simulink model "NewModuleTry_cs"  (Simulink 8.4)
settings: Solver=ode5  SolverMode=SingleTasking  StartTime=0.0  StopTime=inf  FixedStep=1/100  RelTol=1e-3
PreLoadFcn:
  | mbxruntime.callbacks.PreLoadFcn(bdroot);
PostLoadFcn:
  | mbxruntime.callbacks.PostLoadFcn(bdroot);
InitFcn:
  | mbxruntime.callbacks.InitFcn(bdroot);
StartFcn:
  | mbxruntime.callbacks.StartFcn(bdroot);
StopFcn:
  | mbxruntime.callbacks.StopFcn(bdroot);
undefined symbols (not defined in the file or in its folder): dfreq, gray, InitImageOutputDir, Rec, SDTV, strel
libraries: simulink x41, PreScanSimulinkLibrary x15, visiontextngfix x15, simulink_extras x12, visionconversions x3, PreScanUsefulBlocks x3, visionsinks x2, visionstatistics x1, visionmorphops x1, visionanalysis x1, simulink_need_slupdate x1
(part 4 of 7)

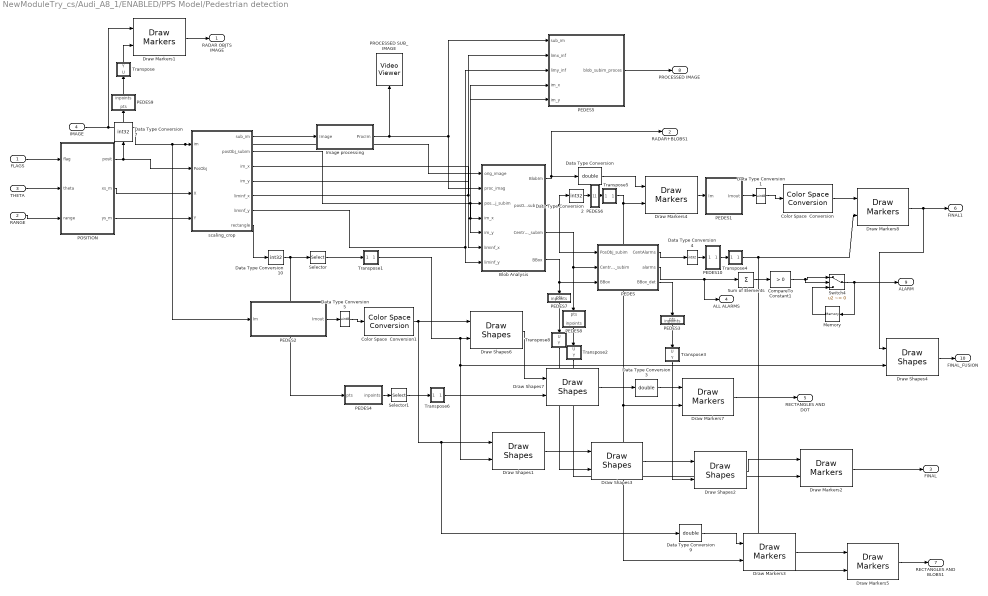
== system NewModuleTry_cs/Audi_A8_1/ENABLED/PPS Model/Pedestrian detection ==
  FLAGS : Inport  OutDataTypeStr=boolean
  RANGE : Inport  Port=2  PortDimensions=TISdet
  THETA : Inport  Port=3
  IMAGE : Inport  Port=4  OutDataTypeStr=uint8  PortDimensions=[375 500]
  Blob Analysis : Subsystem
  Color Space  Conversion : visionconversions/Color Space  Conversion  conversion=Obsolete  conversionActive=Y'CbCr to R'G'B'  wp_str=D65  rec=Rec. 601 (SDTV)  sys=1125/60/2:1  imagePorts=One multidimensional signal
  Color Space  Conversion1 : visionconversions/Color Space  Conversion  conversion=Obsolete  conversionActive=Y'CbCr to R'G'B'  wp_str=D65  rec=Rec. 601 (SDTV)  sys=1125/60/2:1  imagePorts=One multidimensional signal
  CompareTo Constant1 : simulink/Logic and Bit Operations/Compare To Constant  relop=>  const=0  OutDataTypeStr=uint8
  Data Type Conversion : DataTypeConversion  OutDataTypeStr=double
  Data Type Conversion1 : DataTypeConversion  OutDataTypeStr=uint8
  Data Type Conversion{2,4,7,10} (4 alike) : DataTypeConversion  OutDataTypeStr=int32
  Data Type Conversion3 : DataTypeConversion  OutDataTypeStr=double
  Data Type Conversion5 : DataTypeConversion  OutDataTypeStr=uint8
  Data Type Conversion9 : DataTypeConversion  OutDataTypeStr=double
  Draw Markers1 : visiontextngfix/Draw Markers  shape=Circle  size=6  fill=on  fillClrSource=Specify via dialog  display=White  intensity=200  color=[200 255 100]  opacity=1  viewport=Entire image  antialiasing=on  inType=Obsolete  imagePorts=One multidimensional signal  prodOutputMode=Binary point scaling  prodOutputWordLength=32  prodOutputFracLength=14  memoryMode=Specify word length  memoryWordLength=16  memoryFracLength=14  roundingMode=Floor  overflowMode=off
  Draw Markers2 : visiontextngfix/Draw Markers  shape=X-mark  size=3  fill=on  fillClrSource=Specify via dialog  display=White  intensity=200  color=[200 255 100]  opacity=0.9  viewport=Entire image  antialiasing=on  inType=Obsolete  imagePorts=One multidimensional signal  prodOutputMode=Binary point scaling  prodOutputWordLength=32  prodOutputFracLength=14  memoryMode=Specify word length  memoryWordLength=16  memoryFracLength=14  roundingMode=Floor  overflowMode=off
  Draw Markers3 : visiontextngfix/Draw Markers  shape=Circle  size=6  fill=on  fillClrSource=Specify via dialog  display=White  intensity=200  color=[255 0 0]  opacity=0.9  viewport=Entire image  antialiasing=on  inType=Obsolete  imagePorts=One multidimensional signal  prodOutputMode=Binary point scaling  prodOutputWordLength=32  prodOutputFracLength=14  memoryMode=Specify word length  memoryWordLength=16  memoryFracLength=14  roundingMode=Floor  overflowMode=off
  Draw Markers4 : visiontextngfix/Draw Markers  shape=Circle  size=6  fill=on  fillClrSource=Specify via dialog  display=White  intensity=200  color=[200 255 100]  opacity=0.9  viewport=Entire image  antialiasing=on  inType=Obsolete  imagePorts=One multidimensional signal  prodOutputMode=Binary point scaling  prodOutputWordLength=32  prodOutputFracLength=14  memoryMode=Specify word length  memoryWordLength=16  memoryFracLength=14  roundingMode=Floor  overflowMode=off
  Draw Markers5 : visiontextngfix/Draw Markers  shape=Circle  size=6  fill=on  fillClrSource=Specify via dialog  display=User-specified value  intensity=200  color=[255 0 0]  opacity=1  viewport=Entire image  antialiasing=on  inType=Obsolete  imagePorts=One multidimensional signal  prodOutputMode=Binary point scaling  prodOutputWordLength=32  prodOutputFracLength=14  memoryMode=Specify word length  memoryWordLength=16  memoryFracLength=14  roundingMode=Floor  overflowMode=off
  Draw Markers7 : visiontextngfix/Draw Markers  shape=Circle  size=6  fill=on  fillClrSource=Specify via dialog  display=White  intensity=200  color=[200 255 100]  opacity=0.9  viewport=Entire image  antialiasing=on  inType=Obsolete  imagePorts=One multidimensional signal  prodOutputMode=Binary point scaling  prodOutputWordLength=32  prodOutputFracLength=14  memoryMode=Specify word length  memoryWordLength=16  memoryFracLength=14  roundingMode=Floor  overflowMode=off
  Draw Markers8 : visiontextngfix/Draw Markers  shape=Circle  size=6  fill=on  fillClrSource=Specify via dialog  display=User-specified value  intensity=200  color=[255 0 0]  opacity=1  viewport=Entire image  antialiasing=on  inType=Obsolete  imagePorts=One multidimensional signal  prodOutputMode=Binary point scaling  prodOutputWordLength=32  prodOutputFracLength=14  memoryMode=Specify word length  memoryWordLength=16  memoryFracLength=14  roundingMode=Floor  overflowMode=off
  Draw Shapes1 : visiontextngfix/Draw Shapes  shape=Rectangles  fill=off  lineWidth=1  fillClrSource=Specify via dialog  display=White  intensity=200  color=[255 0 0]  opacity=0.5  viewport=Entire image  antialiasing=off  inType=Obsolete  imagePorts=One multidimensional signal  prodOutputMode=Binary point scaling  prodOutputWordLength=32  prodOutputFracLength=14  memoryMode=Specify word length  memoryWordLength=16  memoryFracLength=14  roundingMode=Floor  overflowMode=off
  Draw Shapes2 : visiontextngfix/Draw Shapes  shape=Rectangles  fill=on  lineWidth=1  fillClrSource=Specify via dialog  display=White  intensity=200  color=[255 0 0]  opacity=0.5  viewport=Entire image  antialiasing=off  inType=Obsolete  imagePorts=One multidimensional signal  prodOutputMode=Binary point scaling  prodOutputWordLength=32  prodOutputFracLength=14  memoryMode=Specify word length  memoryWordLength=16  memoryFracLength=14  roundingMode=Floor  overflowMode=off
  Draw Shapes3 : visiontextngfix/Draw Shapes  shape=Rectangles  fill=off  lineWidth=1  fillClrSource=Specify via dialog  display=User-specified value  intensity=200  color=[255 0 0]  opacity=0.5  viewport=Entire image  antialiasing=off  inType=Obsolete  imagePorts=One multidimensional signal  prodOutputMode=Binary point scaling  prodOutputWordLength=32  prodOutputFracLength=14  memoryMode=Specify word length  memoryWordLength=16  memoryFracLength=14  roundingMode=Floor  overflowMode=off
  Draw Shapes4 : visiontextngfix/Draw Shapes  shape=Rectangles  fill=off  lineWidth=1  fillClrSource=Specify via dialog  display=White  intensity=200  color=[255 0 0]  opacity=0.5  viewport=Entire image  antialiasing=off  inType=Obsolete  imagePorts=One multidimensional signal  prodOutputMode=Binary point scaling  prodOutputWordLength=32  prodOutputFracLength=14  memoryMode=Specify word length  memoryWordLength=16  memoryFracLength=14  roundingMode=Floor  overflowMode=off
  Draw Shapes6 : visiontextngfix/Draw Shapes  shape=Rectangles  fill=off  lineWidth=1  fillClrSource=Specify via dialog  display=User-specified value  intensity=200  color=[255 0 0]  opacity=0.6  viewport=Entire image  antialiasing=off  inType=Obsolete  imagePorts=One multidimensional signal  prodOutputMode=Binary point scaling  prodOutputWordLength=32  prodOutputFracLength=14  memoryMode=Specify word length  memoryWordLength=16  memoryFracLength=15  roundingMode=Floor  overflowMode=off
  Draw Shapes7 : visiontextngfix/Draw Shapes  shape=Rectangles  fill=on  lineWidth=1  fillClrSource=Specify via dialog  display=White  intensity=200  color=[255 0 0]  opacity=0.5  viewport=Entire image  antialiasing=off  inType=Obsolete  imagePorts=One multidimensional signal  prodOutputMode=Binary point scaling  prodOutputWordLength=32  prodOutputFracLength=14  memoryMode=Specify word length  memoryWordLength=16  memoryFracLength=14  roundingMode=Floor  overflowMode=off
  Image processing : Subsystem
  Memory : Memory
  PEDES : MATLAB Function  TreatAsAtomicUnit=on
  PEDES1 : MATLAB Function  TreatAsAtomicUnit=on
  PEDES10 : MATLAB Function  TreatAsAtomicUnit=on
  PEDES2 : MATLAB Function  TreatAsAtomicUnit=on
  PEDES3 : MATLAB Function  TreatAsAtomicUnit=on
  PEDES4 : MATLAB Function  TreatAsAtomicUnit=on
  PEDES5 : MATLAB Function  TreatAsAtomicUnit=on
  PEDES6 : MATLAB Function  TreatAsAtomicUnit=on
  PEDES7 : MATLAB Function  TreatAsAtomicUnit=on
  PEDES8 : MATLAB Function  TreatAsAtomicUnit=on
  PEDES9 : MATLAB Function  TreatAsAtomicUnit=on
  POSITION : MATLAB Function  TreatAsAtomicUnit=on
  PROCESSED SUB_IMAGE : visionsinks/Video Viewer  inputType=Obsolete7b  imagePorts=One multidimensional signal  useColorMap=off  colormapValue=gray(256)  specRange=off  minInputVal=0  maxInputVal=255  FigPos=[662 991 500 324]  AxisZoom=on  trueSizedOnce=off  OpenAtMdlStart=on  DefaultConfigurationName=vipscopes.VideoViewerScopeCfg
  Selector : Selector  InputPortWidth=4  Indices=[2, 1, 4, 3]
  Selector1 : Selector  InputPortWidth=4  Indices=[2, 1, 4, 3]
  Sum of Elements : Sum  Inputs=+
  Switch4 : Switch  Criteria=u2 ~= 0
  Transpose : Subsystem
  Transpose1 : Subsystem
  Transpose2 : Subsystem
  Transpose3 : Subsystem
  Transpose4 : Subsystem
  Transpose5 : Subsystem
  Transpose6 : Subsystem
  Transpose8 : Subsystem
  scaling_crop : MATLAB Function  TreatAsAtomicUnit=on
  RADAR OBJTS IMAGE : Outport
  RADAR+BLOBS1 : Outport  Port=2
  FINAL : Outport  Port=3
  ALL ALARMS : Outport  Port=4
  RECTANGLES AND DOT : Outport  Port=5
  FINAL1 : Outport  Port=6
  RECTANGLES AND BLOBS1 : Outport  Port=7
  PROCESSED IMAGE : Outport  Port=8
  ALARM : Outport  Port=9
  FINAL_FUSION : Outport  Port=10
  wires:
  THETA/1 -> POSITION/2(theta)
  FLAGS/1 -> POSITION/1(flag)
  RANGE/1 -> POSITION/3(range)
  Blob Analysis/1(BlobIm) -> RADAR+BLOBS1/1, Data Type Conversion/1
  Blob Analysis/3(Centroid_subim) -> PEDES/2(Centroid_subim), PEDES8/1(pts)
  PEDES/2(alarms) -> ALL ALARMS/1, Sum of Elements/1
  PEDES/1(CentAlarms) -> Data Type Conversion4/1
  Blob Analysis/4(BBox) -> PEDES/3(BBox), PEDES7/1(pts)
  Draw Markers4/1 -> PEDES1/1(Im)
  Data Type Conversion4/1 -> PEDES10/1(pts)
  Color Space  Conversion/1 -> Draw Markers8/1
  PEDES1/1(Imout) -> Data Type Conversion1/1
  Data Type Conversion1/1 -> Color Space  Conversion/1
  Data Type Conversion2/1 -> PEDES6/1(pts)
  Switch4/1 -> Memory/1, ALARM/1
  Memory/1 -> Switch4/3
  Sum of Elements/1 -> CompareTo Constant1/1
  CompareTo Constant1/1 -> Switch4/1, Switch4/2
  Blob Analysis/2(posObj_subim1) -> Data Type Conversion2/1, PEDES/1(PosObj_subim)
  scaling_crop/6(liminf_y) -> PEDES5/3(limy_inf), Blob Analysis/7(liminf_y)
  scaling_crop/7(rectangle) -> Data Type Conversion10/1
  PEDES2/1(Imout) -> Data Type Conversion5/1
  Data Type Conversion5/1 -> Color Space  Conversion1/1
  Color Space  Conversion1/1 -> Draw Shapes6/1, Data Type Conversion9/1, Draw Shapes1/1
  Draw Shapes6/1 -> Draw Shapes7/1
  Draw Shapes7/1 -> Data Type Conversion3/1
  Draw Markers7/1 -> RECTANGLES AND DOT/1
  Draw Shapes1/1 -> Draw Shapes3/1
  Draw Shapes3/1 -> Draw Shapes2/1
  Draw Shapes2/1 -> Draw Markers2/1
  Draw Markers3/1 -> Draw Markers5/1
  Draw Markers5/1 -> RECTANGLES AND BLOBS1/1
  PEDES5/1(blob_subim_proces) -> PROCESSED IMAGE/1
  Draw Markers8/1 -> FINAL1/1, Draw Shapes4/1
  Draw Shapes4/1 -> FINAL_FUSION/1
  Data Type Conversion7/1 -> PEDES9/1(pts)
  POSITION/2(xs_m) -> scaling_crop/3(X)
  Draw Markers1/1 -> RADAR OBJTS IMAGE/1
  POSITION/3(ys_m) -> scaling_crop/4(Y)
  POSITION/1(posit) -> scaling_crop/2(PosObj), Data Type Conversion7/1
  IMAGE/1 -> Blob Analysis/1(orig_image), scaling_crop/1(im), PEDES2/1(Im), Draw Markers1/1
  scaling_crop/1(sub_im) -> Image processing/1(Image)
  scaling_crop/2(posObj_subim) -> Blob Analysis/3(posObj_subim)
  scaling_crop/3(im_x) -> PEDES5/4(im_x), Blob Analysis/4(im_x)
  scaling_crop/4(im_y) -> PEDES5/5(im_y), Blob Analysis/5(im_y)
  scaling_crop/5(liminf_x) -> Blob Analysis/6(liminf_x), PEDES5/2(limx_inf)
  PEDES/3(BBox_det) -> PEDES3/1(pts)
  Draw Markers2/1 -> FINAL/1
  Image processing/1(ProcIm) -> PEDES5/1(sub_im), Blob Analysis/2(proc_imag), PROCESSED SUB_IMAGE/1
  Data Type Conversion/1 -> Draw Markers4/1
  Data Type Conversion9/1 -> Draw Markers3/1
  Data Type Conversion3/1 -> Draw Markers7/1
  Transpose/1(Y) -> Draw Markers1/2
  Transpose1/1(Y) -> Draw Shapes4/2, Draw Shapes1/2, Draw Shapes6/2
  Selector/1 -> Transpose1/1(U)
  Transpose4/1(Y) -> Draw Markers8/2, Draw Markers5/2
  Data Type Conversion10/1 -> Selector/1, PEDES4/1(pts)
  PEDES4/1(inpoints) -> Selector1/1
  Selector1/1 -> Transpose6/1(U)
  Transpose6/1(Y) -> Draw Shapes7/2
  PEDES6/1(inpoints) -> Transpose5/1(U)
  Transpose5/1(Y) -> Draw Markers7/2, Draw Markers3/2, Draw Markers4/2
  PEDES9/1(inpoints) -> Transpose/1(U)
  PEDES10/1(inpoints) -> Transpose4/1(U)
  Transpose3/1(Y) -> Draw Shapes2/2
  Transpose2/1(Y) -> Draw Markers2/2
  Transpose8/1(Y) -> Draw Shapes3/2
  PEDES7/1(inpoints) -> Transpose8/1(U)
  PEDES8/1(inpoints) -> Transpose2/1(U)
  PEDES3/1(inpoints) -> Transpose3/1(U)

== system NewModuleTry_cs/Audi_A8_1/ENABLED/PPS Model/Radar detection ==
  EGO_velocity [m/s] : Inport
  EGO_yaw_rate_[deg/s] : Inport  Port=2
  TIS_range [m] : Inport  Port=3  PortDimensions=TISdet
  TIS_rangedot [m/s] : Inport  Port=4  PortDimensions=TISdet
  TIS_theta [deg] : Inport  Port=5  PortDimensions=TISdet
  ind flag : Inport  Port=6
  Abs : Abs
  Bend road segment : Subsystem  TreatAsAtomicUnit=on
  Compare To Constant : simulink/Logic and Bit Operations/Compare To Constant  relop=<=  const=MaxSpeed/3.6  OutDataTypeStr=uint8
  Constant : Constant  Value=2.0
  Constant2 : Constant  Value=1.0
  Data Store Read : DataStoreRead  DataStoreName=full_brake  SampleTime=1/Mainfreq
  Data Type Conversion : DataTypeConversion  OutDataTypeStr=double
  EGO_velocity [m/s]1 : InportShadow
  EGO_yaw_rate_[deg/s]_1 : InportShadow  Port=2
  If : If  IfExpression=u1 > 1  SampleTime=1/TISfreq
  Logical Operator1 : Logic  Operator=NOT  AllPortsSameDT=off  OutDataTypeStr=boolean
  Merge{1..4} (4 alike) : Merge
  Radians to Degrees : simulink_extras/Transformations/Radians to Degrees
  Straight road segment : Subsystem  TreatAsAtomicUnit=on
  Switch : Switch  Criteria=u2 > Threshold
  TIS1 Sorting  Fun : Subsystem
  change lane : Logic  Inputs=3  AllPortsSameDT=off  OutDataTypeStr=boolean
  change lane1 : Logic  Inputs=3  AllPortsSameDT=off  OutDataTypeStr=boolean
  change lane2 : Logic  Inputs=3  AllPortsSameDT=off  OutDataTypeStr=boolean
  TTC_min_out : Outport
  all_flags0.6 : Outport  Port=2
  all_flags1.6 : Outport  Port=3
  all_flags2 : Outport  Port=4
  all_range [m] : Outport  Port=5
  all_theta [deg] : Outport  Port=6
  wires:
  TIS_range [m]/1 -> TIS1 Sorting  Fun/1(TIS1range [m])
  TIS_rangedot [m/s]/1 -> TIS1 Sorting  Fun/2(TIS1rangedot [m/s])
  TIS_theta [deg]/1 -> TIS1 Sorting  Fun/3(TIS1theta [deg])
  EGO_yaw_rate_[deg/s]/1 -> Abs/1
  If/1 -> Bend road segment/Action
  Abs/1 -> If/1
  TIS1 Sorting  Fun/1(TIS1_RANGE [m]) -> Bend road segment/1(TIS_range [m]), Straight road segment/1(TIS_range [m]1), all_range [m]/1
  TIS1 Sorting  Fun/2(TIS1_RANGEDOT [m/s]) -> Bend road segment/2(TIS_rangedot [m/s]), Straight road segment/2(TIS_rangedot [m/s]1)
  TIS1 Sorting  Fun/3(TIS1_THETA [rad]) -> Bend road segment/3(TIS_theta [deg]), Straight road segment/3(TIS_theta [deg]1), Radians to Degrees/1
  If/2 -> Straight road segment/Action
  Constant2/1 -> Bend road segment/4(TTCdem1), Straight road segment/4(TTCdem1)
  Constant/1 -> Bend road segment/5(TTCdem2), Straight road segment/5(TTCdem2)
  EGO_velocity [m/s]/1 -> Bend road segment/6(EGO_velocity [m/s]1), Straight road segment/6(EGO_velocity [m/s])
  EGO_yaw_rate_[deg/s]_1/1 -> Bend road segment/7(EGO_yaw_rate_[deg/s])
  ind flag/1 -> Data Type Conversion/1
  Bend road segment/2(all_flags_0.6) -> Merge2/1
  Straight road segment/2(all_flags_0.6) -> Merge2/2
  Straight road segment/3(all_flags1.6) -> Merge3/2
  Bend road segment/3(all_flags_1.6) -> Merge3/1
  Radians to Degrees/1 -> all_theta [deg]/1
  Data Type Conversion/1 -> Logical Operator1/1
  Straight road segment/4(TTC_out) -> Merge1/2
  Bend road segment/4(TTC_out) -> Merge1/1
  Merge1/1 -> TTC_min_out/1
  Bend road segment/1(all_flags_2) -> Merge4/1
  Straight road segment/1(all_flags_2) -> Merge4/2
  Merge4/1 -> change lane/2
  Logical Operator1/1 -> change lane/1, change lane2/1, change lane1/1
  Merge3/1 -> change lane1/2
  Merge2/1 -> change lane2/2
  change lane/1 -> all_flags2/1
  change lane2/1 -> Switch/2, Switch/1
  Switch/1 -> all_flags0.6/1
  EGO_velocity [m/s]1/1 -> Compare To Constant/1
  Compare To Constant/1 -> change lane2/3, change lane1/3, change lane/3
  change lane1/1 -> all_flags1.6/1
  Data Store Read/1 -> Switch/3

== system NewModuleTry_cs/Audi_A8_1/ENABLED/PPS Model/Rate transition from TIS to camera ==
  In1 : Inport
  In2 : Inport  Port=2
  In3 : Inport  Port=3
  Rate Transition1 : RateTransition  Integrity=off  Deterministic=off  X0=zeros(TISdet,1)  OutPortSampleTime=1/Camfreq
  Rate Transition2 : RateTransition  Integrity=off  Deterministic=off  X0=zeros(TISdet,1)  OutPortSampleTime=1/Camfreq
  Rate Transition3 : RateTransition  Integrity=off  Deterministic=off  X0=zeros(TISdet,1)  OutPortSampleTime=1/Camfreq
  Out1 : Outport
  Out2 : Outport  Port=2
  Out3 : Outport  Port=3
  wires:
  In1/1 -> Rate Transition3/1
  In2/1 -> Rate Transition1/1
  In3/1 -> Rate Transition2/1
  Rate Transition3/1 -> Out1/1
  Rate Transition1/1 -> Out2/1
  Rate Transition2/1 -> Out3/1

== system NewModuleTry_cs/Audi_A8_1/ENABLED/PPS Model/Rate transition from main freq to TIS freq ==
  In1 : Inport
  In2 : Inport  Port=2
  Rate Transition1 : RateTransition  Integrity=off  Deterministic=off  OutPortSampleTime=1/TISfreq
  Rate Transition2 : RateTransition  Integrity=off  Deterministic=off  OutPortSampleTime=1/TISfreq
  Out1 : Outport
  Out2 : Outport  Port=2
  wires:
  Rate Transition1/1 -> Out2/1
  In2/1 -> Rate Transition1/1
  In1/1 -> Rate Transition2/1
  Rate Transition2/1 -> Out1/1

== system NewModuleTry_cs/Audi_A8_1/ENABLED/PathFollower_1/CTRL REFERENCES ==
  note: REFERENCE POSITION BASED POSITION CTRL
  Pos x,y,Y [m,m,rad] : Inport
  Position Preview Distance [m] : Inport  Port=2
  TrajOffset [m,m,rad] : Inport  Port=3
  ActorOffset_Left(+) / Right(-)_[m] : Inport  Port=4
  Calculate Preview Point (pvp) by extrapolating current Vehicle Position (p0) with Preview Distance and Vehicle Orientation : Subsystem
  Demux : Demux  Outputs=[2 2]
  Demux1 : Demux  Outputs=2
  Demux2 : Demux  Outputs=2
  Find Reference Point (pref) on Trajectory closest to PVP Point (pvp) : Subsystem
      mask Display:
      | port_label('input',1,'pvp [m,m]');
      | port_label('input',2,'TrajOffset_x_y_Y [m,m,rad]');
      | port_label('input',3,'ActorOffset_Left_Right [m]');
      | port_label('input',4,'p0 [m,m,rad]');
      | port_label('output',1,'pref [m,m]');
      | port_label('output',2,'Actor_traj_distance [m]');
      | port_label('output',3,'Actor_traj_angle [m]');
  Mux1 : Mux  Inputs=2
  Reshape : Reshape  OutputDimensionality=Customize  OutputDimensions=[2,2]
  Selector1 : Selector  InputPortWidth=3  Indices=[1 2]
  Terminator : Terminator
  Terminator1 : Terminator
  Terminator2 : Terminator
  Vector Concatenate : Concatenate
  pvp  [m,m] : Outport
  pref_pvp [m,m] : Outport  Port=2
  pref_0 [m,m] : Outport  Port=3
  Actor/Traj_distance [m] : Outport  Port=4
  Actor/Traj_angle [deg] : Outport  Port=5
  wires:
  Demux1/2 -> Terminator2/1
  Demux2/2 -> Terminator1/1
  Demux1/1 -> Actor/Traj_distance [m]/1
  Demux2/1 -> Actor/Traj_angle [deg]/1
  Find Reference Point (pref) on Trajectory closest to PVP Point (pvp)/1(Out1) -> Demux/1
  Reshape/1 -> Find Reference Point (pref) on Trajectory closest to PVP Point (pvp)/1(In1)
  Vector Concatenate/1 -> Reshape/1
  Mux1/1 -> Vector Concatenate/2, pvp  [m,m]/1
  Pos x,y,Y [m,m,rad]/1 -> Calculate Preview Point (pvp) by extrapolating current Vehicle Position (p0) with Preview Distance and Vehicle Orientation/2(x,y,Y Demux [m,m,rad]), Find Reference Point (pref) on Trajectory closest to PVP Point (pvp)/4(In4), Selector1/1
  Calculate Preview Point (pvp) by extrapolating current Vehicle Position (p0) with Preview Distance and Vehicle Orientation/1(x_glob_PVD) -> Mux1/1
  Calculate Preview Point (pvp) by extrapolating current Vehicle Position (p0) with Preview Distance and Vehicle Orientation/3(Y [rad]) -> Terminator/1
  Position Preview Distance [m]/1 -> Calculate Preview Point (pvp) by extrapolating current Vehicle Position (p0) with Preview Distance and Vehicle Orientation/1(Preview Distance)
  Demux/2 -> pref_pvp [m,m]/1
  Demux/1 -> pref_0 [m,m]/1
  Calculate Preview Point (pvp) by extrapolating current Vehicle Position (p0) with Preview Distance and Vehicle Orientation/2(y_glob_PVD) -> Mux1/2
  TrajOffset [m,m,rad]/1 -> Find Reference Point (pref) on Trajectory closest to PVP Point (pvp)/2(In2)  "L6"
  ActorOffset_Left(+) / Right(-)_[m]/1 -> Find Reference Point (pref) on Trajectory closest to PVP Point (pvp)/3(In3)
  Selector1/1 -> Vector Concatenate/1
  Find Reference Point (pref) on Trajectory closest to PVP Point (pvp)/2(Out2) -> Demux1/1
  Find Reference Point (pref) on Trajectory closest to PVP Point (pvp)/3(Out3) -> Demux2/1

== system NewModuleTry_cs/Audi_A8_1/ENABLED/PathFollower_1/Calculate shifted p0 wrt COG ==
  position x,y,Y [m,m,deg] : Inport
  Constant1 : Constant  Value=XShifting_wrt_COG
  Degrees to Radians : simulink_extras/Transformations/Degrees to Radians
  Demux1 : Demux  Outputs=3
  Fcn : Fcn  Expr=u(2)*cos(u(1))
  Fcn1 : Fcn  Expr=u(2)*sin(u(1))
  Mux1 : Mux  Inputs=3
  Mux2 : Mux  Inputs=2
  Sum : Sum  Inputs=|++
  Sum1 : Sum  Inputs=|++
  position x,y,Y [m,m,rad] : Outport
  wires:
  Sum/1 -> Mux1/1
  Sum1/1 -> Mux1/2
  Demux1/1 -> Sum/1
  Demux1/3 -> Degrees to Radians/1
  Degrees to Radians/1 -> Mux2/1, Mux1/3
  Mux2/1 -> Fcn/1, Fcn1/1
  Fcn/1 -> Sum/2
  Fcn1/1 -> Sum1/2
  Demux1/2 -> Sum1/1
  position x,y,Y [m,m,deg]/1 -> Demux1/1
  Mux1/1 -> position x,y,Y [m,m,rad]/1
  Constant1/1 -> Mux2/2

== system NewModuleTry_cs/Audi_A8_1/ENABLED/PathFollower_1/DELTA CTRL ==
  note: POSITION BASED STEERWHEEL CONTROL
  p0 : Inport
  pvp : Inport  Port=2
  pref_pvp : Inport  Port=3
  pref0 : Inport  Port=4
  Calculate preview angle : Subsystem
      mask Display:
      | port_label('input',1,'pvp [m,m]');
      | port_label('input',2,'pref [m,m]');
      | port_label('input',3,'p0 [m,m]');
      | port_label('output',1,'angle [rad]');
  Divide2 : Product
  Divide4 : Product
  Error check : Subsystem
  Goto Tag Visibility : GotoTagVisibility  GotoTag=pref0
  Goto Tag Visibility1 : GotoTagVisibility  GotoTag=p0
  Radians to Degrees1 : simulink_extras/Transformations/Radians to Degrees
  Selector2 : Selector  InputPortWidth=3  Indices=[1 2]
  Steering angle  velocity dependent : Lookup  InputValues=[0 18 40 60 70 80 90 100 110]  Table=[16.5 16.5 28 44.5 55 60.5 60.5 60.5 60.5]
  Steering angle preview  distance dependent : Lookup  InputValues=[0 1 4 5 6 7 8 9 10 11 20 21]  Table=[1.5 1.5 1 1 1 1 1 1 0.9 0.9 0.8 0.8]
  These limits are  the vehicle maximum  steering wheel angle : Saturate  UpperLimit=720  LowerLimit=-720
  TunableSteering Gain : Gain  Gain=TunableSteeringGain
  sign1 : Gain  Gain=3.6
  delta_steerwheel [deg] : Outport
  tag scope: p0=scoped, pref0=scoped
  wires:
  Calculate preview angle/1(Out1) -> Radians to Degrees1/1
  Selector2/1 -> Calculate preview angle/3(In3)
  p0/1 -> Selector2/1, [p0]
  pvp/1 -> Calculate preview angle/1(In1)
  pref_pvp/1 -> Calculate preview angle/2(In2)
  Radians to Degrees1/1 -> Divide2/2
  These limits are  the vehicle maximum  steering wheel angle/1 -> delta_steerwheel [deg]/1
  pref0/1 -> [pref0]
  sign1/1 -> Steering angle  velocity dependent/1
  [v_actual] -> sign1/1
  Steering angle  velocity dependent/1 -> Divide2/1
  Divide4/1 -> TunableSteering Gain/1
  Divide2/1 -> Divide4/1
  Steering angle preview  distance dependent/1 -> Divide4/2
  [PreviewDistance] -> Steering angle preview  distance dependent/1
  TunableSteering Gain/1 -> These limits are  the vehicle maximum  steering wheel angle/1

== system NewModuleTry_cs/Audi_A8_1/ENABLED/PathFollower_1/THROTTLE CTRL ==
  v_actual [m/s] : Inport
  Desired Velocity [m/s] : Inport  Port=2
  Initial Velocity [m/s] : Inport  Port=3
  Demux : Demux  Outputs=3
  GearNormal : Constant
  "GearNormal " : Constant
  If Desired Velocity = 0 : Subsystem  TreatAsAtomicUnit=on
  If Desired Velocity ~= 0 : Subsystem  TreatAsAtomicUnit=on
  Merge : Merge
  Mux : Mux  Inputs=3
  Mux2 : Mux  Inputs=3
  Sum4 : Sum  Inputs=|+-
  if : If  IfExpression=u1 == 0
  throttle [%] : Outport
  brake pressure [bar] : Outport  Port=2
  v0 [m/s] : Outport  Port=3
  Auto_GearShift : Outport  Port=4
  wires:
  v_actual [m/s]/1 -> Sum4/2
  If Desired Velocity ~= 0/3(Auto_GearShift) -> Mux2/3
  If Desired Velocity ~= 0/2(brake pressure [bar]) -> Mux2/2
  If Desired Velocity ~= 0/1(throttle [%]) -> Mux2/1
  if/1 -> If Desired Velocity = 0/Action
  if/2 -> If Desired Velocity ~= 0/Action
  If Desired Velocity = 0/3(Auto_GearShift) -> Mux/3
  "GearNormal "/1 -> If Desired Velocity ~= 0/1(In1)
  Demux/3 -> Auto_GearShift/1
  Demux/2 -> brake pressure [bar]/1
  Demux/1 -> throttle [%]/1
  Mux/1 -> Merge/1
  Mux2/1 -> Merge/2
  If Desired Velocity = 0/2(brake pressure [bar]) -> Mux/2
  If Desired Velocity = 0/1(throttle [%]) -> Mux/1
  Merge/1 -> Demux/1
  GearNormal/1 -> If Desired Velocity = 0/1(In1)
  Initial Velocity [m/s]/1 -> v0 [m/s]/1
  Desired Velocity [m/s]/1 -> Sum4/1, if/1
  Sum4/1 -> If Desired Velocity ~= 0/2(Desired Velocity [m/s])

== system NewModuleTry_cs/Audi_A8_1/ENABLED/SELF_Demux/compas converter ==
  rotz [rad] : Inport
  cart2compas : Subsystem
  rad2deg : Gain  Gain=180/pi
  heading [deg] : Outport
  wires:
  rad2deg/1 -> cart2compas/1(Angle [deg])
  rotz [rad]/1 -> rad2deg/1
  cart2compas/1(heading [deg]) -> heading [deg]/1

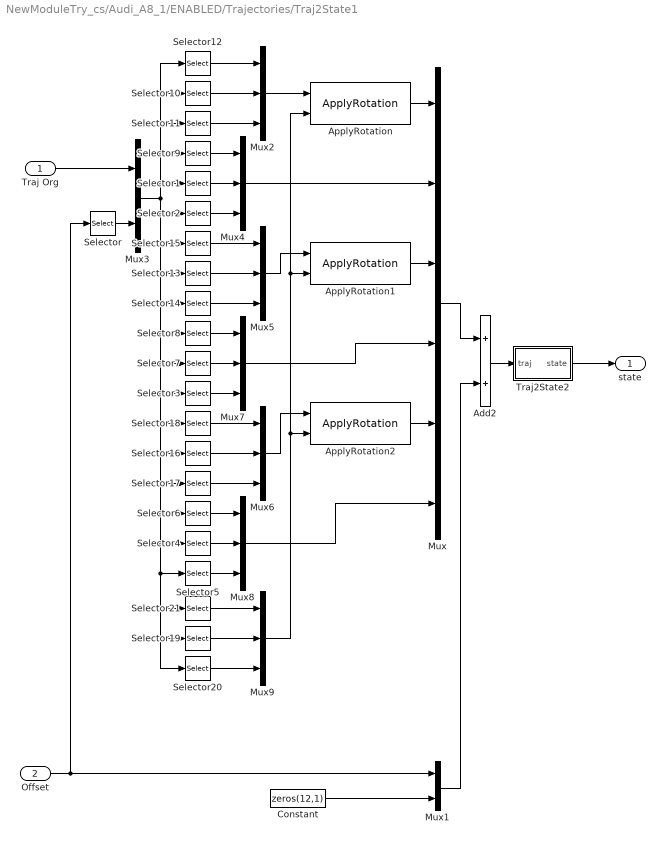
== system NewModuleTry_cs/Audi_A8_1/ENABLED/Trajectories/Traj2State1 ==
  Traj Org : Inport
  Offset : Inport  Port=2
  Add2 : Sum
  ApplyRotation : PreScanSimulinkLibrary/ApplyRotation
  ApplyRotation1 : PreScanSimulinkLibrary/ApplyRotation
  ApplyRotation2 : PreScanSimulinkLibrary/ApplyRotation
  Constant : Constant  Value=zeros(12,1)
  Mux : Mux  Inputs=6
  Mux1 : Mux  Inputs=2
  Mux{2,4..9} (7 alike) : Mux  Inputs=3
  Mux3 : Mux  Inputs=2
  Selector : Selector  InputPortWidth=6  Indices=[4 5 6]
  Selector1 : Selector  InputPortWidth=21  Indices=[5]
  Selector10 : Selector  InputPortWidth=21  Indices=[2]
  Selector11 : Selector  InputPortWidth=21  Indices=[3]
  Selector12 : Selector  InputPortWidth=21  Indices=[1]
  Selector13 : Selector  InputPortWidth=21  Indices=[8]
  Selector14 : Selector  InputPortWidth=21  Indices=[9]
  Selector15 : Selector  InputPortWidth=21  Indices=[7]
  Selector16 : Selector  InputPortWidth=21  Indices=[14]
  Selector17 : Selector  InputPortWidth=21  Indices=[15]
  Selector18 : Selector  InputPortWidth=21  Indices=[13]
  Selector19 : Selector  InputPortWidth=21  Indices=[20]
  Selector2 : Selector  InputPortWidth=21  Indices=[6]
  Selector20 : Selector  InputPortWidth=21  Indices=[21]
  Selector21 : Selector  InputPortWidth=21  Indices=[19]
  Selector3 : Selector  InputPortWidth=21  Indices=[12]
  Selector4 : Selector  InputPortWidth=21  Indices=[17]
  Selector5 : Selector  InputPortWidth=21  Indices=[18]
  Selector6 : Selector  InputPortWidth=21  Indices=[16]
  Selector7 : Selector  InputPortWidth=21  Indices=[11]
  Selector8 : Selector  InputPortWidth=21  Indices=[10]
  Selector9 : Selector  InputPortWidth=21  Indices=[4]
  Traj2State2 : Subsystem
  state : Outport
  wires:
  Mux9/1 -> ApplyRotation2/2, ApplyRotation1/2, ApplyRotation/2
  Selector20/1 -> Mux9/3
  Selector19/1 -> Mux9/2
  Selector21/1 -> Mux9/1
  Selector5/1 -> Mux8/3
  Selector4/1 -> Mux8/2
  Selector6/1 -> Mux8/1
  Mux8/1 -> Mux/6
  Mux6/1 -> ApplyRotation2/1
  Mux7/1 -> Mux/4
  ApplyRotation2/1 -> Mux/5
  Selector3/1 -> Mux7/3
  Selector7/1 -> Mux7/2
  Selector8/1 -> Mux7/1
  Mux4/1 -> Mux/2
  Mux5/1 -> ApplyRotation1/1
  ApplyRotation1/1 -> Mux/3
  Mux2/1 -> ApplyRotation/1
  ApplyRotation/1 -> Mux/1
  Selector2/1 -> Mux4/3
  Selector1/1 -> Mux4/2
  Selector9/1 -> Mux4/1
  Selector17/1 -> Mux6/3
  Selector16/1 -> Mux6/2
  Selector18/1 -> Mux6/1
  Selector14/1 -> Mux5/3
  Selector13/1 -> Mux5/2
  Selector15/1 -> Mux5/1
  Selector11/1 -> Mux2/3
  Selector10/1 -> Mux2/2
  Selector12/1 -> Mux2/1
  Mux3/1 -> Selector8/1, Selector7/1, Selector3/1, Selector18/1, Selector16/1, Selector17/1, Selector6/1, Selector20/1, Selector19/1, Selector21/1, Selector5/1, Selector4/1, Selector14/1, Selector13/1, Selector15/1, Selector2/1, Selector1/1, Selector9/1, Selector12/1, Selector10/1, Selector11/1
  Mux1/1 -> Add2/2
  Constant/1 -> Mux1/2
  Add2/1 -> Traj2State2/1(traj)
  Selector/1 -> Mux3/2
  Traj Org/1 -> Mux3/1
  Offset/1 -> Mux1/1, Selector/1
  Mux/1 -> Add2/1
  Traj2State2/1(state) -> state/1

== system NewModuleTry_cs/Audi_A8_1/ENABLED/Trajectories/TrajCoGOffset ==
  State In : Inport
  Add : Sum  Inputs=+-+
  Add1 : Sum
  ApplyRotation : PreScanSimulinkLibrary/ApplyRotation
  ApplyRotation1 : PreScanSimulinkLibrary/ApplyRotation
  CoG Offset : Constant  Value=[0 0 CoGOffsetZ]
  Degrees to Radians : simulink_extras/Transformations/Degrees to Radians
  Demux1 : Demux  Outputs=[3 3 3]
  Mux : Mux  Inputs=[3 3 3]
  Orientation : Constant  Value=[InitRoll InitPitch 0]
  State Out : Outport
  wires:
  State In/1 -> Demux1/1
  Demux1/1 -> Add/1
  Add/1 -> Mux/1
  Demux1/3 -> Mux/3, Add1/2
  Mux/1 -> State Out/1
  Demux1/2 -> Mux/2
  Orientation/1 -> Degrees to Radians/1
  ApplyRotation/1 -> Add/3
  ApplyRotation1/1 -> Add/2
  Add1/1 -> ApplyRotation/2
  CoG Offset/1 -> ApplyRotation1/1, ApplyRotation/1
  Degrees to Radians/1 -> Add1/1, ApplyRotation1/2

== system NewModuleTry_cs/Audi_A8_1/ENABLED/Trajectories/Trajectory_1 ==
  From Workspace : FromWorkspace  VariableName=trajectory  SampleTime=TimeStep  OutputAfterFinalValue=Holding final value
  From Workspace1 : FromWorkspace  VariableName=trajectory  SampleTime=TimeStep  OutputAfterFinalValue=Setting to zero
  Mux : Mux  Inputs=2
  Selector1 : Selector  InputPortWidth=24  Indices=[7:18]
  Selector9 : Selector  InputPortWidth=24  Indices=[1:6]
  trajectory : Outport
  wires:
  From Workspace/1 -> Selector9/1
  From Workspace1/1 -> Selector1/1
  Mux/1 -> trajectory/1
  Selector9/1 -> Mux/1
  Selector1/1 -> Mux/2

== system NewModuleTry_cs/Audi_A8_1/ENABLED/V2X_244_Generic_Filter/Filter ==
  In : Inport
  Filter : MATLAB Function  TreatAsAtomicUnit=on
  Zero : Constant  Value=0  OutDataTypeStr=Bus: PRESCAN_V2X_USER_GENERIC_MESSAGE
  Out : Outport
  wires:
  Zero/1 -> Filter/2(z)
  Filter/1(y) -> Out/1
  In/1 -> Filter/1(u)

== system NewModuleTry_cs/BMW_Z3_1/ENABLED/Dynamics_Empty/MuxState ==
  note: mode: Dynamics
  note: mode: Positioning
  note: mode: Dynamics
      | VelVEHICLE
      | wrt VEH
  note: AnglesVEHICLE
      | wrtGLOB
  note: For state mode 'Dynamic' positions
      | are not taken into account, as they
      | are computed by integrating velocity.
      | Click annotation for Help.
  x [m] : Inport  SampleTime=TimeStep
  y [m] : Inport  Port=2  SampleTime=TimeStep
  z [m] : Inport  Port=3  SampleTime=TimeStep
  dx [m/s] : Inport  Port=4  SampleTime=TimeStep
  dy [m/s] : Inport  Port=5  SampleTime=TimeStep
  dz [m/s] : Inport  Port=6  SampleTime=TimeStep
  R [rad] : Inport  Port=7  SampleTime=TimeStep
  P [rad] : Inport  Port=8  SampleTime=TimeStep
  Y [rad] : Inport  Port=9  SampleTime=TimeStep
  Constant : Constant  DisableCoverage=on  Value=positioningmode
  Discrete-Time Integrator : DiscreteIntegrator  SampleTime=TimeStep
  Ground : Ground
  Ground1 : Ground
  Mux1 : Mux  Inputs=[3 3]
  Mux2 : Mux  Inputs=3
  Mux3 : Mux  Inputs=3
  Mux4 : Mux  Inputs=3
  Mux5 : Mux  Inputs=[3 3]
  Mux6 : Mux  Inputs=[6 3]
  Switch : Switch  Threshold=0.5
  Transformation_BODY2GLOBAL : PreScanSimulinkLibrary/Simple_Vehicle_Dynamics/Chassis/MuxDynState/Transformation_BODY2GLOBAL
  mux3 : Mux  Inputs=3
  state : Outport
  wires:
  Constant/1 -> Switch/2
  Mux6/1 -> state/1
  Mux4/1 -> Mux1/1
  Mux5/1 -> Switch/3
  Mux1/1 -> Switch/1
  Switch/1 -> Mux6/1  "PosVeh wrt  GLOB"
  P [rad]/1 -> Mux3/2
  R [rad]/1 -> Mux3/1
  dz [m/s]/1 -> Mux2/3
  dy [m/s]/1 -> Mux2/2
  dx [m/s]/1 -> Mux2/1
  z [m]/1 -> Mux4/3
  y [m]/1 -> Mux4/2
  x [m]/1 -> Mux4/1
  Ground1/1 -> mux3/2  "pitch"
  Y [rad]/1 -> mux3/3, Mux3/3  "yaw"
  Mux3/1 -> Mux6/2
  Transformation_BODY2GLOBAL/1 -> Discrete-Time Integrator/1, Mux5/2  "VelVEH wrt  GLOB"
  mux3/1 -> Transformation_BODY2GLOBAL/2
  Ground/1 -> mux3/1  "roll"
  Mux2/1 -> Mux1/2, Transformation_BODY2GLOBAL/1
  Discrete-Time Integrator/1 -> Mux5/1  "PosVEH wrt  GLOB"

== system NewModuleTry_cs/BMW_Z3_1/ENABLED/SELF_Demux/compas converter ==
  rotz [rad] : Inport
  cart2compas : Subsystem
  rad2deg : Gain  Gain=180/pi
  heading [deg] : Outport
  wires:
  rad2deg/1 -> cart2compas/1(Angle [deg])
  rotz [rad]/1 -> rad2deg/1
  cart2compas/1(heading [deg]) -> heading [deg]/1

== system NewModuleTry_cs/BMW_Z3_1/ENABLED/V2X_243_Generic_Filter/Filter ==
  In : Inport
  Filter : MATLAB Function  TreatAsAtomicUnit=on
  Zero : Constant  Value=0  OutDataTypeStr=Bus: PRESCAN_V2X_USER_GENERIC_MESSAGE
  Out : Outport
  wires:
  Zero/1 -> Filter/2(z)
  Filter/1(y) -> Out/1
  In/1 -> Filter/1(u)

== system NewModuleTry_cs/CollisionDetection/DISABLED/GND1/GND_DATA ==
  GND_ObjectID1 : Constant  Value=uint32(0)
  GND_ObjectID2 : Constant  Value=uint32(0)
  buscreator : BusCreator  Inputs=2  OutDataTypeStr=Bus: PRESCAN_COLLISIONDETECTION_DATA  NonVirtualBus=on
  bus : Outport  OutDataTypeStr=Bus: PRESCAN_COLLISIONDETECTION_DATA
  wires:
  GND_ObjectID1/1 -> buscreator/1  "ObjectID1"
  GND_ObjectID2/1 -> buscreator/2  "ObjectID2"
  buscreator/1 -> bus/1

== system NewModuleTry_cs/CollisionDetection/DISABLED/GND1/GND_HEADER ==
  GND_valid : Constant  Value=boolean(0)
  buscreator : BusCreator  Inputs=1  OutDataTypeStr=Bus: PRESCAN_HEADER  NonVirtualBus=on
  bus : Outport  OutDataTypeStr=Bus: PRESCAN_HEADER
  wires:
  GND_valid/1 -> buscreator/1  "valid"
  buscreator/1 -> bus/1

== system NewModuleTry_cs/Male_RegularAni_1/ENABLED/Animation/animation mode ==
  vel : Inport
  Data Type Conversion : DataTypeConversion  OutDataTypeStr=double
  Fcn : Fcn  Expr=sqrt(u(1)^2+u(2)^2+u(3)^2)
  Running : simulink/Logic and Bit Operations/Compare To Constant  relop=>=  const=MWS  OutDataTypeStr=uint8  ZeroCross=off
  Sum : Sum  Inputs=|++
  Walking : simulink/Logic and Bit Operations/Compare To Zero  relop=~=  OutDataTypeStr=uint8  ZeroCross=off
  mode : Outport
  wires:
  vel/1 -> Fcn/1
  Sum/1 -> Data Type Conversion/1
  Walking/1 -> Sum/1
  Running/1 -> Sum/2
  Fcn/1 -> Walking/1, Running/1
  Data Type Conversion/1 -> mode/1

== system NewModuleTry_cs/Male_RegularAni_1/ENABLED/Animation/elapsed track ==
  vel : Inport
  Discrete-Time Integrator : DiscreteIntegrator  SampleTime=-1
  Fcn : Fcn  Expr=sqrt(u(1)^2 + u(2)^2 + u(3)^2)
  s : Outport
  wires:
  Fcn/1 -> Discrete-Time Integrator/1
  vel/1 -> Fcn/1
  Discrete-Time Integrator/1 -> s/1

== system NewModuleTry_cs/Male_RegularAni_1/ENABLED/SELF_Demux/compas converter ==
  rotz [rad] : Inport
  cart2compas : Subsystem
  rad2deg : Gain  Gain=180/pi
  heading [deg] : Outport
  wires:
  rad2deg/1 -> cart2compas/1(Angle [deg])
  rotz [rad]/1 -> rad2deg/1
  cart2compas/1(heading [deg]) -> heading [deg]/1

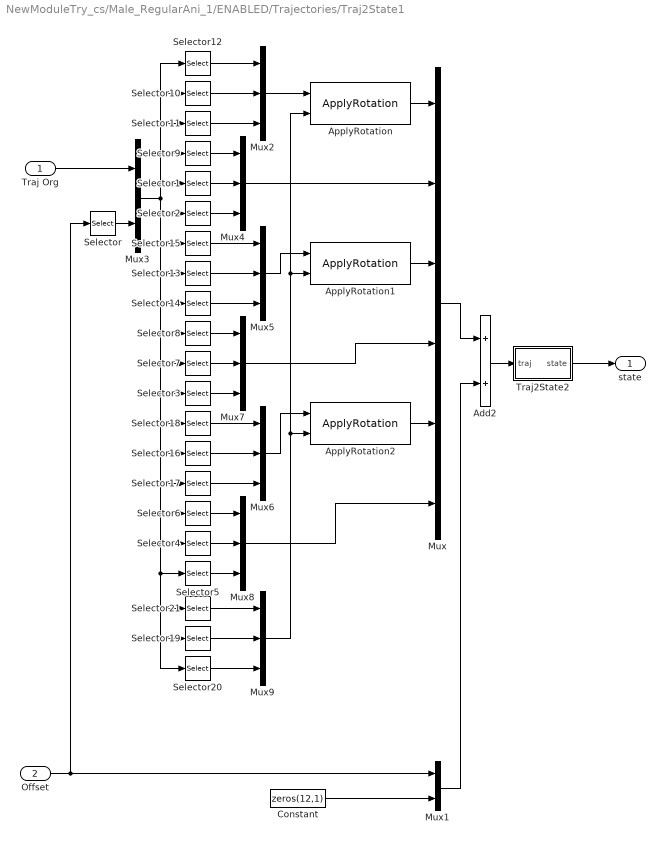
== system NewModuleTry_cs/Male_RegularAni_1/ENABLED/Trajectories/Traj2State1 ==
  Traj Org : Inport
  Offset : Inport  Port=2
  Add2 : Sum
  ApplyRotation : PreScanSimulinkLibrary/ApplyRotation
  ApplyRotation1 : PreScanSimulinkLibrary/ApplyRotation
  ApplyRotation2 : PreScanSimulinkLibrary/ApplyRotation
  Constant : Constant  Value=zeros(12,1)
  Mux : Mux  Inputs=6
  Mux1 : Mux  Inputs=2
  Mux{2,4..9} (7 alike) : Mux  Inputs=3
  Mux3 : Mux  Inputs=2
  Selector : Selector  InputPortWidth=6  Indices=[4 5 6]
  Selector1 : Selector  InputPortWidth=21  Indices=[5]
  Selector10 : Selector  InputPortWidth=21  Indices=[2]
  Selector11 : Selector  InputPortWidth=21  Indices=[3]
  Selector12 : Selector  InputPortWidth=21  Indices=[1]
  Selector13 : Selector  InputPortWidth=21  Indices=[8]
  Selector14 : Selector  InputPortWidth=21  Indices=[9]
  Selector15 : Selector  InputPortWidth=21  Indices=[7]
  Selector16 : Selector  InputPortWidth=21  Indices=[14]
  Selector17 : Selector  InputPortWidth=21  Indices=[15]
  Selector18 : Selector  InputPortWidth=21  Indices=[13]
  Selector19 : Selector  InputPortWidth=21  Indices=[20]
  Selector2 : Selector  InputPortWidth=21  Indices=[6]
  Selector20 : Selector  InputPortWidth=21  Indices=[21]
  Selector21 : Selector  InputPortWidth=21  Indices=[19]
  Selector3 : Selector  InputPortWidth=21  Indices=[12]
  Selector4 : Selector  InputPortWidth=21  Indices=[17]
  Selector5 : Selector  InputPortWidth=21  Indices=[18]
  Selector6 : Selector  InputPortWidth=21  Indices=[16]
  Selector7 : Selector  InputPortWidth=21  Indices=[11]
  Selector8 : Selector  InputPortWidth=21  Indices=[10]
  Selector9 : Selector  InputPortWidth=21  Indices=[4]
  Traj2State2 : Subsystem
  state : Outport
  wires:
  Mux9/1 -> ApplyRotation2/2, ApplyRotation1/2, ApplyRotation/2
  Selector20/1 -> Mux9/3
  Selector19/1 -> Mux9/2
  Selector21/1 -> Mux9/1
  Selector5/1 -> Mux8/3
  Selector4/1 -> Mux8/2
  Selector6/1 -> Mux8/1
  Mux8/1 -> Mux/6
  Mux6/1 -> ApplyRotation2/1
  Mux7/1 -> Mux/4
  ApplyRotation2/1 -> Mux/5
  Selector3/1 -> Mux7/3
  Selector7/1 -> Mux7/2
  Selector8/1 -> Mux7/1
  Mux4/1 -> Mux/2
  Mux5/1 -> ApplyRotation1/1
  ApplyRotation1/1 -> Mux/3
  Mux2/1 -> ApplyRotation/1
  ApplyRotation/1 -> Mux/1
  Selector2/1 -> Mux4/3
  Selector1/1 -> Mux4/2
  Selector9/1 -> Mux4/1
  Selector17/1 -> Mux6/3
  Selector16/1 -> Mux6/2
  Selector18/1 -> Mux6/1
  Selector14/1 -> Mux5/3
  Selector13/1 -> Mux5/2
  Selector15/1 -> Mux5/1
  Selector11/1 -> Mux2/3
  Selector10/1 -> Mux2/2
  Selector12/1 -> Mux2/1
  Mux3/1 -> Selector8/1, Selector7/1, Selector3/1, Selector18/1, Selector16/1, Selector17/1, Selector6/1, Selector20/1, Selector19/1, Selector21/1, Selector5/1, Selector4/1, Selector14/1, Selector13/1, Selector15/1, Selector2/1, Selector1/1, Selector9/1, Selector12/1, Selector10/1, Selector11/1
  Mux1/1 -> Add2/2
  Constant/1 -> Mux1/2
  Add2/1 -> Traj2State2/1(traj)
  Selector/1 -> Mux3/2
  Traj Org/1 -> Mux3/1
  Offset/1 -> Mux1/1, Selector/1
  Mux/1 -> Add2/1
  Traj2State2/1(state) -> state/1

== system NewModuleTry_cs/Male_RegularAni_1/ENABLED/Trajectories/TrajCoGOffset ==
  State In : Inport
  Add : Sum  Inputs=+-+
  Add1 : Sum
  ApplyRotation : PreScanSimulinkLibrary/ApplyRotation
  ApplyRotation1 : PreScanSimulinkLibrary/ApplyRotation
  CoG Offset : Constant  Value=[0 0 CoGOffsetZ]
  Degrees to Radians : simulink_extras/Transformations/Degrees to Radians
  Demux1 : Demux  Outputs=[3 3 3]
  Mux : Mux  Inputs=[3 3 3]
  Orientation : Constant  Value=[InitRoll InitPitch 0]
  State Out : Outport
  wires:
  State In/1 -> Demux1/1
  Demux1/1 -> Add/1
  Add/1 -> Mux/1
  Demux1/3 -> Mux/3, Add1/2
  Mux/1 -> State Out/1
  Demux1/2 -> Mux/2
  Orientation/1 -> Degrees to Radians/1
  ApplyRotation/1 -> Add/3
  ApplyRotation1/1 -> Add/2
  Add1/1 -> ApplyRotation/2
  CoG Offset/1 -> ApplyRotation1/1, ApplyRotation/1
  Degrees to Radians/1 -> Add1/1, ApplyRotation1/2

== system NewModuleTry_cs/Male_RegularAni_1/ENABLED/Trajectories/Trajectory_2 ==
  From Workspace : FromWorkspace  VariableName=trajectory  SampleTime=TimeStep  OutputAfterFinalValue=Holding final value
  From Workspace1 : FromWorkspace  VariableName=trajectory  SampleTime=TimeStep  OutputAfterFinalValue=Setting to zero
  Mux : Mux  Inputs=2
  Selector1 : Selector  InputPortWidth=24  Indices=[7:18]
  Selector9 : Selector  InputPortWidth=24  Indices=[1:6]
  trajectory : Outport
  wires:
  From Workspace/1 -> Selector9/1
  From Workspace1/1 -> Selector1/1
  Mux/1 -> trajectory/1
  Selector9/1 -> Mux/1
  Selector1/1 -> Mux/2

== system NewModuleTry_cs/TIS_1/DISABLED/GND1/GND_DATA ==
  GND_ActiveBeamID : Constant  Value=uint32(0)
  GND_Alpha : Constant  Value=0
  GND_Beta : Constant  Value=0
  GND_DopplerVelocity : Constant  Value=0
  GND_DopplerVelocityRotationX : Constant  Value=0
  GND_DopplerVelocityRotationY : Constant  Value=0
  GND_DopplerVelocityRotationZ : Constant  Value=0
  GND_DopplerVelocityTranslationX : Constant  Value=0
  GND_DopplerVelocityTranslationY : Constant  Value=0
  GND_DopplerVelocityTranslationZ : Constant  Value=0
  GND_EnergyLoss : Constant  Value=0
  GND_Phi : Constant  Value=0
  GND_Range : Constant  Value=0
  GND_TargetID : Constant  Value=uint32(0)
  GND_TargetTypeID : Constant  Value=uint32(0)
  GND_Theta : Constant  Value=0
  buscreator : BusCreator  Inputs=16  OutDataTypeStr=Bus: PRESCAN_SCANNERSENSOR_DATA  NonVirtualBus=on
  bus : Outport  OutDataTypeStr=Bus: PRESCAN_SCANNERSENSOR_DATA
  wires:
  GND_ActiveBeamID/1 -> buscreator/1  "ActiveBeamID"
  GND_Range/1 -> buscreator/2  "Range"
  GND_DopplerVelocity/1 -> buscreator/3  "DopplerVelocity"
  GND_Theta/1 -> buscreator/4  "Theta"
  GND_Phi/1 -> buscreator/5  "Phi"
  GND_TargetID/1 -> buscreator/6  "TargetID"
  GND_TargetTypeID/1 -> buscreator/7  "TargetTypeID"
  GND_EnergyLoss/1 -> buscreator/8  "EnergyLoss"
  GND_Alpha/1 -> buscreator/9  "Alpha"
  GND_Beta/1 -> buscreator/10  "Beta"
  GND_DopplerVelocityTranslationX/1 -> buscreator/11  "DopplerVelocityTranslationX"
  GND_DopplerVelocityTranslationY/1 -> buscreator/12  "DopplerVelocityTranslationY"
  GND_DopplerVelocityTranslationZ/1 -> buscreator/13  "DopplerVelocityTranslationZ"
  GND_DopplerVelocityRotationX/1 -> buscreator/14  "DopplerVelocityRotationX"
  GND_DopplerVelocityRotationY/1 -> buscreator/15  "DopplerVelocityRotationY"
  GND_DopplerVelocityRotationZ/1 -> buscreator/16  "DopplerVelocityRotationZ"
  buscreator/1 -> bus/1

== system NewModuleTry_cs/TIS_1/DISABLED/GND1/GND_HEADER ==
  GND_valid : Constant  Value=boolean(0)
  buscreator : BusCreator  Inputs=1  OutDataTypeStr=Bus: PRESCAN_HEADER  NonVirtualBus=on
  bus : Outport  OutDataTypeStr=Bus: PRESCAN_HEADER
  wires:
  GND_valid/1 -> buscreator/1  "valid"
  buscreator/1 -> bus/1

== system NewModuleTry_cs/TIS_2/DISABLED/GND1/GND_DATA ==
  GND_ActiveBeamID : Constant  Value=uint32(0)
  GND_Alpha : Constant  Value=0
  GND_Beta : Constant  Value=0
  GND_DopplerVelocity : Constant  Value=0
  GND_DopplerVelocityRotationX : Constant  Value=0
  GND_DopplerVelocityRotationY : Constant  Value=0
  GND_DopplerVelocityRotationZ : Constant  Value=0
  GND_DopplerVelocityTranslationX : Constant  Value=0
  GND_DopplerVelocityTranslationY : Constant  Value=0
  GND_DopplerVelocityTranslationZ : Constant  Value=0
  GND_EnergyLoss : Constant  Value=0
  GND_Phi : Constant  Value=0
  GND_Range : Constant  Value=0
  GND_TargetID : Constant  Value=uint32(0)
  GND_TargetTypeID : Constant  Value=uint32(0)
  GND_Theta : Constant  Value=0
  buscreator : BusCreator  Inputs=16  OutDataTypeStr=Bus: PRESCAN_SCANNERSENSOR_DATA  NonVirtualBus=on
  bus : Outport  OutDataTypeStr=Bus: PRESCAN_SCANNERSENSOR_DATA
  wires:
  GND_ActiveBeamID/1 -> buscreator/1  "ActiveBeamID"
  GND_Range/1 -> buscreator/2  "Range"
  GND_DopplerVelocity/1 -> buscreator/3  "DopplerVelocity"
  GND_Theta/1 -> buscreator/4  "Theta"
  GND_Phi/1 -> buscreator/5  "Phi"
  GND_TargetID/1 -> buscreator/6  "TargetID"
  GND_TargetTypeID/1 -> buscreator/7  "TargetTypeID"
  GND_EnergyLoss/1 -> buscreator/8  "EnergyLoss"
  GND_Alpha/1 -> buscreator/9  "Alpha"
  GND_Beta/1 -> buscreator/10  "Beta"
  GND_DopplerVelocityTranslationX/1 -> buscreator/11  "DopplerVelocityTranslationX"
  GND_DopplerVelocityTranslationY/1 -> buscreator/12  "DopplerVelocityTranslationY"
  GND_DopplerVelocityTranslationZ/1 -> buscreator/13  "DopplerVelocityTranslationZ"
  GND_DopplerVelocityRotationX/1 -> buscreator/14  "DopplerVelocityRotationX"
  GND_DopplerVelocityRotationY/1 -> buscreator/15  "DopplerVelocityRotationY"
  GND_DopplerVelocityRotationZ/1 -> buscreator/16  "DopplerVelocityRotationZ"
  buscreator/1 -> bus/1

== system NewModuleTry_cs/TIS_2/DISABLED/GND1/GND_HEADER ==
  GND_valid : Constant  Value=boolean(0)
  buscreator : BusCreator  Inputs=1  OutDataTypeStr=Bus: PRESCAN_HEADER  NonVirtualBus=on
  bus : Outport  OutDataTypeStr=Bus: PRESCAN_HEADER
  wires:
  GND_valid/1 -> buscreator/1  "valid"
  buscreator/1 -> bus/1

== system NewModuleTry_cs/Audi_A8_1/ENABLED/Dynamics_Simple/Chassis/Bicycle_model_[XYZ] ==
  DeltaWheel_[rad] : Inport
  zFront_[m]_dzFront_[ms-1] : Inport  Port=2  PortDimensions=2
  zRear_[m]_dzRear_[ms-1] : Inport  Port=3  PortDimensions=2
  BrakePressure_[bar] : Inport  Port=4
  DriveTorque_[Nm] : Inport  Port=5
  v0_[ms-1] : Inport  Port=6
  |vx|_[ms-1] : Inport  Port=7
  Fy_rear_[N] : Inport  Port=8
  Fy_front_[N] : Inport  Port=9
  Demux : Demux  Outputs=2
  Demux1 : Demux  Outputs=2
  Fyi --> Fy / Mz : Subsystem
  X_Motion : Subsystem
  Y & Yaw_Motion : Subsystem
  "Z, Pitch_Motion & Roll_Motion" : Subsystem
  |vx|_[ms-1]1 : Outport
  vy_[ms-1] : Outport  Port=2
  vz_[ms-1] : Outport  Port=3
  RollAngle_[rad] : Outport  Port=4
  RollRate_[rads-1] : Outport  Port=5
  YawAngle_[rads-1] : Outport  Port=6
  Vx_[ms-1] : Outport  Port=7
  PitchAngle_[rad] : Outport  Port=8
  YawAngle_[rad] : Outport  Port=9
  ax_[ms-2] : Outport  Port=10
  ay_[ms-2] : Outport  Port=11
  wires:
  Fyi --> Fy / Mz/1(Fy_[N]) -> Y & Yaw_Motion/2(Fy_[N])  "Fy_[N]"
  Fyi --> Fy / Mz/2(Mz_[Nm]) -> Y & Yaw_Motion/3(Mz_[Nm])  "Mz_[Nm]"
  Y & Yaw_Motion/1(|vx|_[ms-1]1) -> |vx|_[ms-1]1/1  "|vx|_[ms-1]"
  Y & Yaw_Motion/2(vy_[ms-1]) -> vy_[ms-1]/1  "vy_[ms-1]"
  Y & Yaw_Motion/5(YawAngle_[rad]) -> YawAngle_[rad]/1  "YawAngle_[rad]"
  v0_[ms-1]/1 -> X_Motion/3(v0_[ms-1])  "v0_[ms-1]"
  BrakePressure_[bar]/1 -> X_Motion/2(BrakePressure_[bar])  "BrakePressure_[bar]"
  DriveTorque_[Nm]/1 -> X_Motion/1(DriveTorque_[Nm])  "DriveTorque_[Nm]"
  X_Motion/2(ax_[ms-2]) -> ax_[ms-2]/1, [ax]  "ax_[ms-2]"
  X_Motion/1(vx_[ms-1]) -> Vx_[ms-1]/1, [vx]  "vx_[ms-1]"
  [ax] -> "Z, Pitch_Motion & Roll_Motion"/3(ax)
  Demux/1 -> "Z, Pitch_Motion & Roll_Motion"/5(zFront_[m])
  Demux/2 -> "Z, Pitch_Motion & Roll_Motion"/6(dzFront_[ms-1])
  Demux1/1 -> "Z, Pitch_Motion & Roll_Motion"/7(zRear_[m])
  Demux1/2 -> "Z, Pitch_Motion & Roll_Motion"/8(dzRear_[ms-1])
  zRear_[m]_dzRear_[ms-1]/1 -> Demux1/1
  zFront_[m]_dzFront_[ms-1]/1 -> Demux/1
  "Z, Pitch_Motion & Roll_Motion"/2(vz_[ms-1]) -> vz_[ms-1]/1  "vz_[ms-1]"
  DeltaWheel_[rad]/1 -> Fyi --> Fy / Mz/1(DeltaWheel_[rad])
  Fy_front_[N]/1 -> Fyi --> Fy / Mz/2(Fy_f_[N])
  Fy_rear_[N]/1 -> Fyi --> Fy / Mz/3(Fy_r_[N])
  |vx|_[ms-1]/1 -> Y & Yaw_Motion/1(|vx|_[ms-1])
  Y & Yaw_Motion/3(ay_[ms-2]) -> [ay], ay_[ms-2]/1  "ay_[ms-2]"
  [ay] -> "Z, Pitch_Motion & Roll_Motion"/4(ay)
  "Z, Pitch_Motion & Roll_Motion"/3(RollAngle_[rad]) -> RollAngle_[rad]/1  "RollAngle_[rad]"
  "Z, Pitch_Motion & Roll_Motion"/4(RollRate_[rads-1]) -> RollRate_[rads-1]/1  "RollRate_[rads-1]"
  [dYaw] -> "Z, Pitch_Motion & Roll_Motion"/2(dYaw)
  [vx] -> "Z, Pitch_Motion & Roll_Motion"/1(vx)
  Y & Yaw_Motion/4(dYawAngle_[rads-1]) -> YawAngle_[rads-1]/1, [dYaw]  "dYawAngle_[rads-1]"
  "Z, Pitch_Motion & Roll_Motion"/1(pitchAngle_[rad]) -> PitchAngle_[rad]/1  "PitchAngle_[rad]"
